simulink model "LQR_sim"  (R2022b)
settings: Solver=VariableStepAuto  StartTime=0.0  StopTime=10  RelTol=1e-3
values from neighbouring files (symbols this model uses):
  A = [-0.051 0 -0.144 -0.056 0 0 0 0 0 0 0 0 ... (169 elements, 13x13)]    [Elicottero.mat]
  B = [0 0 0 0 0 0 0.68 3.043 0 0 0 0 ... (52 elements, 13x4)]    [Elicottero.mat]
undefined symbols (not defined in the file or in its folder): A_k, B_k, BandWidth, C, C_k, D, D_k, K_i_lq, K_s_lq, Qt
libraries: simulink x2
settings Model: Creator=valen  LastModifiedBy=valen
settings ModelReferenceCC: EnableRefExpFcnMdlSchedulingChecks=on

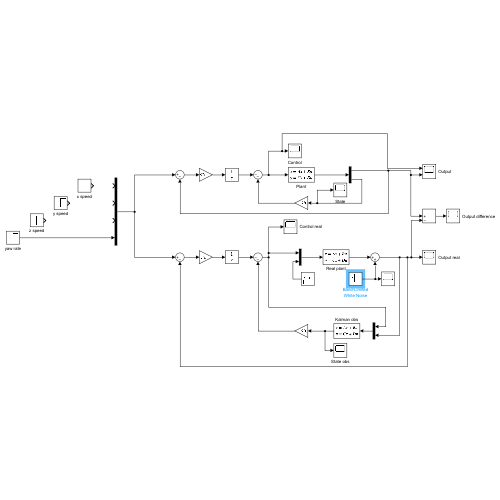
[thumbnail: Simulink's stored preview of the top-level diagram]
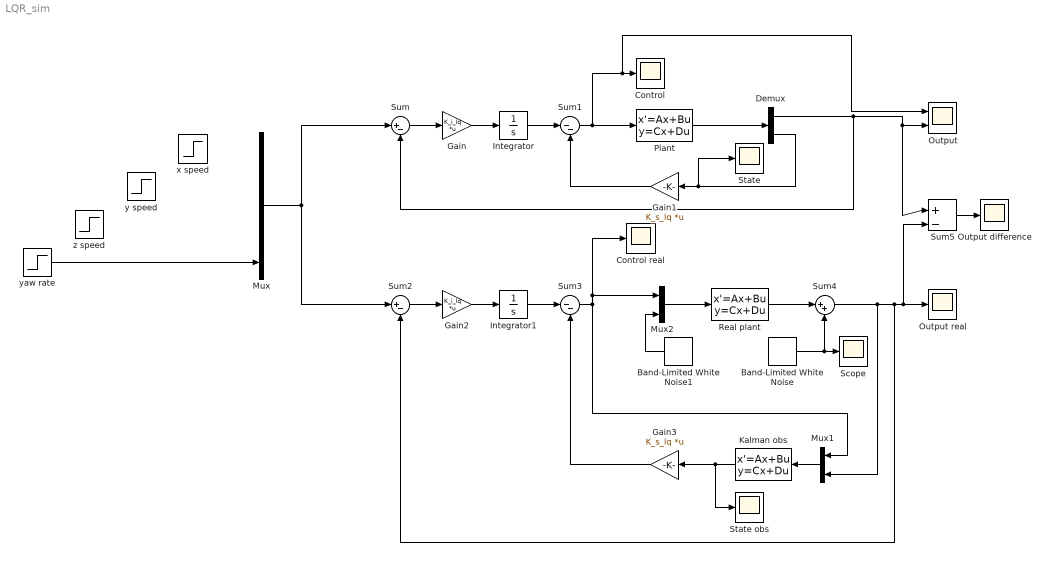
== system LQR_sim ==
  Band-Limited White Noise : simulink/Sources/Band-Limited White Noise  Cov=NoisePower  Ts=1/BandWidth  seed=[23341]
  Band-Limited White Noise1 : simulink/Sources/Band-Limited White Noise  Cov=diag(Qt)  Ts=1/BandWidth  seed=[23341]
  Control : Scope
  Control real : Scope
  Demux : Demux  Outputs=[4, 13]
  Gain : Gain  Gain=K_i_lq  Multiplication=Matrix(K*u)
  Gain1 : Gain  Gain=K_s_lq  Multiplication=Matrix(K*u)
  Gain2 : Gain  Gain=K_i_lq  Multiplication=Matrix(K*u)
  Gain3 : Gain  Gain=K_s_lq  Multiplication=Matrix(K*u)
  Integrator : Integrator
  Integrator1 : Integrator
  Kalman obs : StateSpace  A=A_k  B=B_k  C=C_k  D=D_k  InitialCondition=0
  Mux : Mux
  Mux1 : Mux  Inputs=2
  Mux2 : Mux  Inputs=2
  Output : Scope  NumInputPorts=2
  Output difference : Scope
  Output real : Scope
  Plant : StateSpace  A=A  B=B  C=[C; eye(13)]  D=[D;zeros(13,4)]  InitialCondition=0
  Real plant : StateSpace  A=A  B=[B, eye(13)]  C=C  D=[D, zeros(4,13)]  InitialCondition=rand(13,1).*0.00
  Scope : Scope
  State : Scope
  State obs : Scope
  Sum : Sum  Inputs=|+-
  Sum1 : Sum  Inputs=|--
  Sum2 : Sum  Inputs=|+-
  Sum3 : Sum  Inputs=|--
  Sum4 : Sum  Inputs=|++
  Sum5 : Sum  Inputs=|+-
  x speed : Step  Time=0  SampleTime=0
  y speed : Step  Time=0  SampleTime=0
  yaw rate : Step  Time=0  SampleTime=0
  z speed : Step  Time=0  SampleTime=0
  wires:
  Integrator/1 -> Sum1/1
  Sum1/1 -> Output/1, Control/1, Plant/1
  Gain1/1 -> Sum1/2
  Gain/1 -> Integrator/1
  Sum/1 -> Gain/1
  Demux/2 -> State/1, Gain1/1
  Sum2/1 -> Gain2/1
  Gain2/1 -> Integrator1/1
  Gain3/1 -> Sum3/2
  Sum3/1 -> Mux2/1, Control real/1, Mux1/1
  Integrator1/1 -> Sum3/1
  Kalman obs/1 -> State obs/1, Gain3/1
  Mux1/1 -> Kalman obs/1
  Real plant/1 -> Sum4/1
  Sum4/1 -> Sum2/2, Output real/1, Sum5/2, Mux1/2
  Plant/1 -> Demux/1
  Demux/1 -> Output/2, Sum5/1, Sum/2
  Sum5/1 -> Output difference/1
  Band-Limited White Noise/1 -> Scope/1, Sum4/2
  Mux/1 -> Sum2/1, Sum/1
  Mux2/1 -> Real plant/1
  Band-Limited White Noise1/1 -> Mux2/2
  yaw rate/1 -> Mux/4
